simulink model "observerlinmodel"  (R2016a)
settings: Solver=VariableStepAuto  StartTime=0.0  StopTime=10.0  RelTol=1e-3
values from neighbouring files (symbols this model uses):
  Cs = eye(3)    [Modelscript.m]
  K = place(As,Bs,[-1 -2 -3 -4 -5 -6])    [Modelscript.m]
settings Model: Creator=Lehelxp  LastModifiedBy=Lehelxp

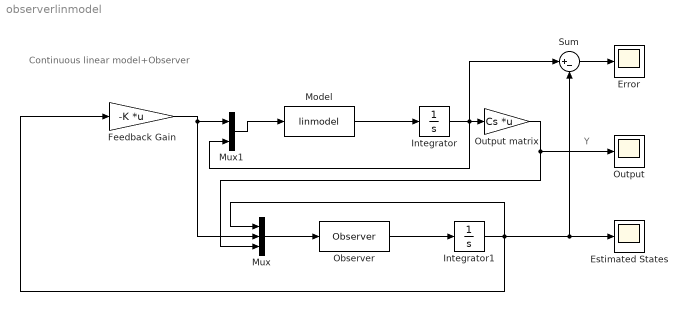
== system observerlinmodel ==
  note: Y
  note: Continuous linear model+Observer
  Error : Scope
  Estimated States : Scope
  Feedback Gain : Gain  Gain=-K  Multiplication=Matrix(K*u) (u vector)
  Integrator : Integrator  InitialCondition=[1 2 0 0 0 0]'
  Integrator1 : Integrator  InitialCondition=[0.1 0.3 0.2 0 0 0]'
  Model : MATLABFcn  MATLABFcn=linmodel  OutputDimensions=6
  Mux : Mux  Inputs=3
  Mux1 : Mux  Inputs=2
  Observer : MATLABFcn  MATLABFcn=Observer  OutputDimensions=6  Output1D=off
  Output : Scope
  Output matrix : Gain  Gain=Cs  Multiplication=Matrix(K*u)
  Sum : Sum  Inputs=|+-
  wires:
  Model/1 -> Integrator/1
  Feedback Gain/1 -> Mux/2, Mux1/1
  Integrator/1 -> Sum/1, Mux1/2, Output matrix/1
  Output matrix/1 -> Mux/3, Output/1
  Mux/1 -> Observer/1
  Observer/1 -> Integrator1/1
  Integrator1/1 -> Estimated States/1, Sum/2, Feedback Gain/1, Mux/1
  Mux1/1 -> Model/1
  Sum/1 -> Error/1
